simulink model "CIE_337_Part_B_Sawtooth"  (R2018b)
settings: Solver=FixedStepAuto  StartTime=0.0  StopTime=2  FixedStep=0.0001  RelTol=1e-3
settings Model: Creator=RAWN  LastModifiedBy=RAWN

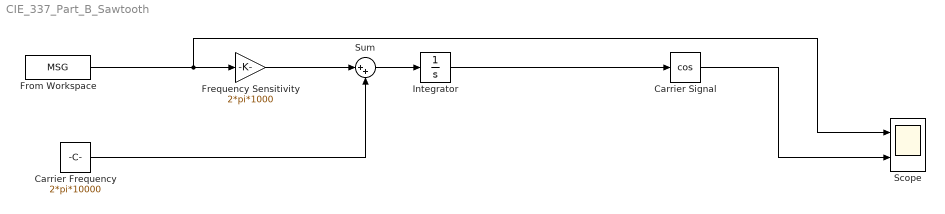
== system CIE_337_Part_B_Sawtooth ==
  Carrier Frequency : Constant  Value=2*pi*10000
  Carrier Signal : Trigonometry  Operator=cos
  Frequency Sensitivity : Gain  Gain=2*pi*1000
  From Workspace : FromWorkspace  VariableName=MSG  SampleTime=0
  Integrator : Integrator
  Scope : Scope  NumInputPorts=2
  Sum : Sum  Inputs=|++
  wires:
  Carrier Signal/1 -> Scope/2
  From Workspace/1 -> Scope/1, Frequency Sensitivity/1
  Carrier Frequency/1 -> Sum/2
  Frequency Sensitivity/1 -> Sum/1
  Sum/1 -> Integrator/1
  Integrator/1 -> Carrier Signal/1
